simulink model "sampleModel1425"  (R2023a)
settings: Solver=VariableStepAuto  StartTime=0.0  StopTime=10.0  RelTol=1e-3
libraries: hdlsllib x10, simulink x3
settings Model: Creator=user1  LastModifiedBy=user1

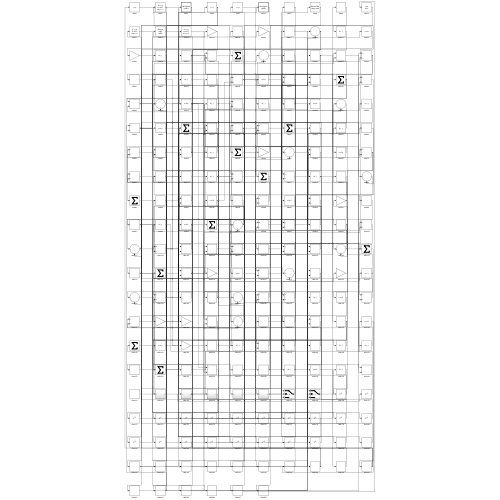
[thumbnail: Simulink's stored preview of the top-level diagram]
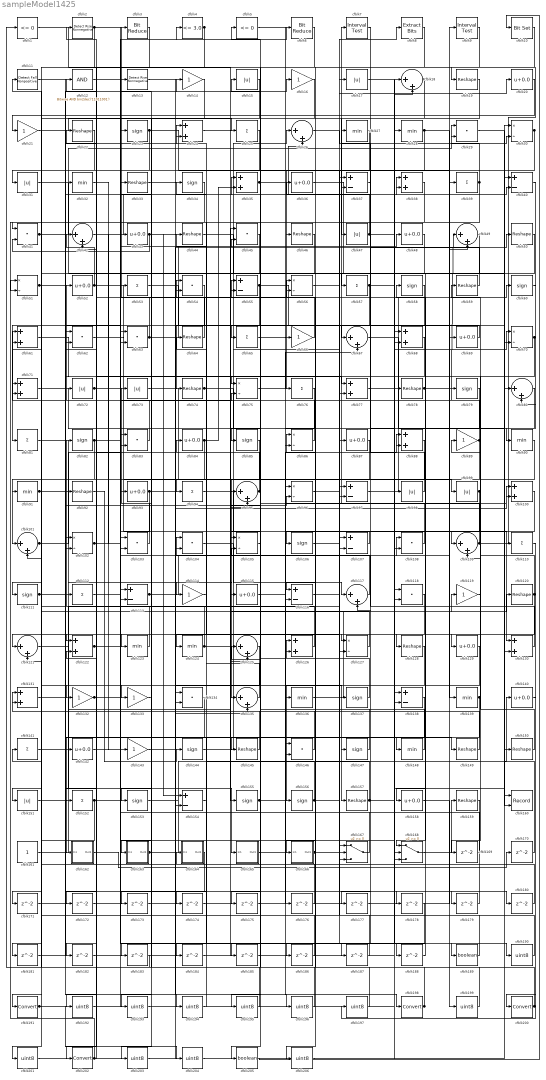
== system sampleModel1425 ==
  cfblk1 : hdlsllib/Logic and Bit Operations/Compare To Zero  relop=<=  OutDataTypeStr=boolean
  cfblk10 : simulink/Logic and Bit Operations/Bit Set  iBit=0
      settings: LibrarySourceBlock=|
      | hdlsllib/Logic and Bit
      | Operations/Bit Set
  cfblk{24,35,38,61,68,71,77,88,100,122,126,130..131} (13 alike) : Sum
  cfblk{18,26,42,49,67,80,95,101,109,117,121,125,135} (13 alike) : Sum  Inputs=|++
  cfblk{30,51,56,70,75,86,96,102,105,127} (10 alike) : Product  Inputs=*/  RndMeth=Zero  SaturateOnIntegerOverflow=on
  cfblk{29,41,45,54,62..63,83,103..104,108,118,134,146} (13 alike) : DotProduct  OutDataTypeStr=Inherit: Inherit via internal rule
  cfblk{23,34,58,60,79,82,85,106,111,137,144,147,153,155..156} (15 alike) : Signum
  cfblk{37,40,55,97,107,113,116,138,154} (9 alike) : Sum  Inputs=+-
  cfblk11 : hdlsllib/Logic and Bit Operations/Detect Fall Nonpositive  vinit=0  OutDataTypeStr=boolean
  cfblk{25,39,53,57,65,76,81,94,110,112,141,152} (12 alike) : Sum  Inputs=+
  cfblk{14,16,21,66,89,114,119,132..133,143} (10 alike) : Gain
  cfblk{20,36,43,48,52,69,84,87,93,115,129,140,142,158} (14 alike) : Bias  Bias=0.0  SaturateOnIntegerOverflow=off
  cfblk12 : simulink/Logic and Bit Operations/Bitwise Operator  logicop=AND  UseBitMask=on  BitMask=bin2dec('11011001')  BitMaskRealWorld=Stored Integer
      settings: LibrarySourceBlock=|
      | hdlsllib/Logic and Bit
      | Operations/Bitwise
      | Operator
  cfblk{19,22,33,44,46,50,59,64,74,78,92,120,128,145,149..150,157,159} (18 alike) : Reshape
  cfblk{27..28,32,90..91,123..124,136,139,148} (10 alike) : MinMax
  cfblk13 : hdlsllib/Logic and Bit Operations/Detect Rise Nonnegative  vinit=0  OutDataTypeStr=boolean
  cfblk{15,17,31,47,72..73,98..99,151} (9 alike) : Abs  SaturateOnIntegerOverflow=off
  cfblk160 : Record  FileSettingsInternal="{\"entries\":[{\"content\":{\"excelSettings\":{\"content\":{},\"type\":\"Streamout.ExcelSettings\"}},\"type\":\"Streamout.FileSettingStorage\",\"uuid\":\"\"}],\"packageUris\":[\"http:\\/\\/schema.mathworks.com\\/mf0\\/streamout_blocks\\/R2020a\"],\"version\":\"1.0\"}"  Layout=[1 1]  SignalsInternal="{\"entries\":[{\"content\":{\"signals\":[{\"content\":{\"blockPath\":[],\"dimensions\":[1],\"domain\":\"\",\"lineColor\":\"#a2142f\",\"plots\":[1],\"port\":1,\"signalID\":401,\"signalName\":\"XY Graph:1\"},\"type\":\"RecordBlkView.Signal\",\"uuid\":\"\"},{\"content\":{\"blockPath\":[],\"dimensions\":[1],\"domain\":\"\",\"lineColor\":\"#139fff\",\"plots\":[1],\"port\":2,\"signalID\":404,\"signalName\":\"XY Graph:2\"},\"type\":\"RecordBlkView.Signal\",\"uuid\":\"\"}]},\"type\":\"RecordBlkView.InputSignals\",\"uuid\":\"\"}],\"packageUris\":[\"http:\\/\\/schema.mathworks.com\\/mf0\\/streamout_blocks\\/R2020a\"],\"version\":\"1.0\"}"  VisualizationBindings="{\"xyplotplugin\":{\"info\":[{\"series\":[{\"bindingParametersList\":[{\"parameter\":\"X-Axis\",\"signalID\":401,\"signalName\":\"XY Graph:1\"},{\"parameter\":\"Y-Axis\",\"signalID\":404,\"signalName\":\"XY Graph:2\"}],\"seriesID\":26922}],\"subplotID\":1}]}}"  CompatibilityTag=XY  st=-1
  cfblk161 : Constant  SampleTime=-1
  cfblk162 : Subsystem
      settings: LibrarySourceBlock=|
      | hdlsllib/Ports &
      | Subsystems/Subsystem
  cfblk163 : Subsystem
      settings: LibrarySourceBlock=|
      | hdlsllib/Ports &
      | Subsystems/Subsystem
  cfblk164 : Subsystem
      settings: LibrarySourceBlock=|
      | hdlsllib/Ports &
      | Subsystems/Subsystem
  cfblk165 : Subsystem
      settings: LibrarySourceBlock=|
      | hdlsllib/Ports &
      | Subsystems/Subsystem
  cfblk166 : Subsystem
      settings: LibrarySourceBlock=|
      | hdlsllib/Ports &
      | Subsystems/Subsystem
  cfblk167 : Switch  SaturateOnIntegerOverflow=off  InputSameDT=off
  cfblk168 : Switch  SaturateOnIntegerOverflow=off  InputSameDT=off
  cfblk{169..188} (20 alike) : Delay  SampleTime=1
  cfblk189 : DataTypeConversion  OutDataTypeStr=boolean  SaturateOnIntegerOverflow=off  RndMeth=Floor
  cfblk{190,192..197,199,201,203..204,206} (12 alike) : DataTypeConversion  OutDataTypeStr=uint8  SaturateOnIntegerOverflow=off  RndMeth=Floor
  cfblk{191,198,200,202} (4 alike) : DataTypeConversion  SaturateOnIntegerOverflow=off  RndMeth=Floor
  cfblk2 : hdlsllib/Logic and Bit Operations/Detect Rise Nonnegative  vinit=0  OutDataTypeStr=boolean
  cfblk205 : DataTypeConversion  OutDataTypeStr=boolean  SaturateOnIntegerOverflow=off  RndMeth=Floor
  cfblk3 : hdlsllib/Logic and Bit Operations/Bit Reduce  mode=AND
  cfblk4 : hdlsllib/Logic and Bit Operations/Compare To Constant  relop=<=  const=3.0  OutDataTypeStr=boolean
  cfblk5 : hdlsllib/Logic and Bit Operations/Compare To Zero  relop=<=  OutDataTypeStr=boolean
  cfblk6 : hdlsllib/Logic and Bit Operations/Bit Reduce  mode=AND
  cfblk7 : hdlsllib/Logic and Bit Operations/Interval Test  IntervalClosedRight=on  uplimit=0.5  IntervalClosedLeft=on  lowlimit=-0.5  OutDataTypeStr=boolean
  cfblk8 : simulink/Logic and Bit Operations/Extract Bits  bitsToExtract=Upper half  numBits=8  bitIdxRange=[0 7]  outScalingMode=Preserve fixed-point scaling
      settings: LibrarySourceBlock=|
      | hdlsllib/Logic and Bit
      | Operations/Extract Bits
  cfblk9 : hdlsllib/Logic and Bit Operations/Interval Test  IntervalClosedRight=on  uplimit=0.5  IntervalClosedLeft=on  lowlimit=-0.5  OutDataTypeStr=boolean
  wires:
  cfblk128/1 -> cfblk157/1
  cfblk144/1 -> cfblk26/1
  cfblk21/1 -> cfblk25/1
  cfblk20/1 -> cfblk21/1
  cfblk166/1(Out1) -> cfblk38/1, cfblk188/1
  cfblk36/1 -> cfblk158/1
  cfblk109/1 -> cfblk19/1, cfblk83/2
  cfblk27/1 -> cfblk31/1
  cfblk32/1 -> cfblk143/1
  cfblk130/1 -> cfblk104/1
  cfblk81/1 -> cfblk165/1(In1)
  cfblk64/1 -> cfblk3/1
  cfblk92/1 -> cfblk144/1
  cfblk87/1 -> cfblk135/1
  cfblk73/1 -> cfblk99/1
  cfblk108/1 -> cfblk7/1
  cfblk123/1 -> cfblk82/1
  cfblk78/1 -> cfblk49/1, cfblk168/1
  cfblk120/1 -> cfblk128/1, cfblk79/1
  cfblk104/1 -> cfblk117/1
  cfblk113/1 -> cfblk9/1, cfblk127/2
  cfblk47/1 -> cfblk36/1, cfblk189/1
  cfblk69/1 -> cfblk65/1
  cfblk18/1 -> cfblk47/1, cfblk193/1
  cfblk147/1 -> cfblk86/1
  cfblk99/1 -> cfblk138/2, cfblk169/1
  cfblk143/1 -> cfblk50/1
  cfblk114/1 -> cfblk44/1
  cfblk70/1 -> cfblk117/2, cfblk129/1
  cfblk153/1 -> cfblk140/1
  cfblk121/1 -> cfblk148/1
  cfblk157/1 -> cfblk70/1, cfblk126/1
  cfblk35/1 -> cfblk26/2, cfblk38/2
  cfblk97/1 -> cfblk39/1
  cfblk54/1 -> cfblk74/1
  cfblk58/1 -> cfblk166/1(In1)
  cfblk139/1 -> cfblk184/1, cfblk195/1
  cfblk149/1 -> cfblk131/1
  cfblk68/1 -> cfblk202/1
  cfblk19/1 -> cfblk105/1
  cfblk129/1 -> cfblk156/1
  cfblk55/1 -> cfblk81/1, cfblk85/1, cfblk108/2
  cfblk161/1 -> cfblk17/1
  cfblk49/1 -> cfblk132/1
  cfblk80/1 -> cfblk147/1
  cfblk84/1 -> cfblk163/1(In1), cfblk35/2
  cfblk41/1 -> cfblk29/1, cfblk75/1
  cfblk116/1 -> cfblk20/1
  cfblk61/1 -> cfblk77/1
  cfblk156/1 -> cfblk87/1, cfblk56/2, cfblk24/2
  cfblk127/1 -> cfblk61/1
  cfblk110/1 -> cfblk200/1
  cfblk71/1 -> cfblk136/1
  cfblk28/1 -> cfblk69/1, cfblk167/3, cfblk177/1
  cfblk15/1 -> cfblk123/1
  cfblk56/1 -> cfblk167/1
  cfblk30/1 -> cfblk76/1, cfblk175/1
  cfblk14/1 -> cfblk121/1
  cfblk63/1 -> cfblk48/1, cfblk2/1
  cfblk77/1 -> cfblk30/1
  cfblk136/1 -> cfblk119/1
  cfblk101/1 -> cfblk23/1, cfblk71/2
  cfblk86/1 -> cfblk61/2
  cfblk165/1(Out1) -> cfblk88/1
  cfblk17/1 -> cfblk109/1
  cfblk62/1 -> cfblk130/1
  cfblk168/1 -> cfblk159/1
  cfblk25/1 -> cfblk111/1
  cfblk39/1 -> cfblk124/1, cfblk51/2, cfblk29/2
  cfblk142/1 -> cfblk16/1
  cfblk112/1 -> cfblk60/1
  cfblk152/1 -> cfblk45/2, cfblk168/3, cfblk201/1
  cfblk91/1 -> cfblk115/1, cfblk179/1
  cfblk52/1 -> cfblk97/2, cfblk42/1
  cfblk103/1 -> cfblk73/1
  cfblk72/1 -> cfblk122/1, cfblk54/2, cfblk185/1
  cfblk83/1 -> cfblk52/1
  cfblk88/1 -> cfblk103/2
  cfblk107/1 -> cfblk106/1
  cfblk126/1 -> cfblk71/1
  cfblk89/1 -> cfblk34/1, cfblk101/1
  cfblk122/1 -> cfblk6/1, cfblk56/1
  cfblk163/1(Out1) -> cfblk45/1, cfblk100/2
  cfblk145/1 -> cfblk22/1
  cfblk117/1 -> cfblk64/1
  cfblk8/1 -> cfblk46/1
  cfblk43/1 -> cfblk67/1, cfblk154/1, cfblk95/1, cfblk41/2, cfblk135/2
  cfblk53/1 -> cfblk80/1
  cfblk7/1 -> cfblk57/1
  cfblk24/1 -> cfblk146/1
  cfblk125/1 -> cfblk151/1
  cfblk155/1 -> cfblk125/1, cfblk100/1
  cfblk38/1 -> cfblk146/2
  cfblk75/1 -> cfblk67/2
  cfblk151/1 -> cfblk96/2
  cfblk31/1 -> cfblk86/2
  cfblk100/1 -> cfblk116/1
  cfblk96/1 -> cfblk107/2
  cfblk60/1 -> cfblk80/2
  cfblk119/1 -> cfblk59/1
  cfblk67/1 -> cfblk160/1
  cfblk131/1 -> cfblk32/1
  cfblk82/1 -> cfblk75/2, cfblk181/1
  cfblk74/1 -> cfblk8/1, cfblk98/1
  cfblk37/1 -> cfblk127/1
  cfblk1/1 -> cfblk155/1
  cfblk134/1 -> cfblk162/1(In1)
  cfblk111/1 -> cfblk149/1, cfblk154/2
  cfblk29/1 -> cfblk130/2
  cfblk23/1 -> cfblk78/1, cfblk139/1, cfblk62/2
  cfblk137/1 -> cfblk83/1
  cfblk4/1 -> cfblk42/2, cfblk192/1
  cfblk124/1 -> cfblk62/1, cfblk120/1
  cfblk94/1 -> cfblk150/1
  cfblk45/1 -> cfblk121/2
  cfblk118/1 -> cfblk191/1
  cfblk159/1 -> cfblk164/1(In1)
  cfblk57/1 -> cfblk77/2, cfblk160/2, cfblk66/1
  cfblk59/1 -> cfblk27/1
  cfblk50/1 -> cfblk142/1
  cfblk26/1 -> cfblk30/2
  cfblk34/1 -> cfblk41/1
  cfblk9/1 -> cfblk145/1
  cfblk42/1 -> cfblk18/2
  cfblk105/1 -> cfblk55/1
  cfblk148/1 -> cfblk92/1
  cfblk76/1 -> cfblk116/2
  cfblk150/1 -> cfblk89/1
  cfblk93/1 -> cfblk134/1, cfblk113/2
  cfblk95/1 -> cfblk94/1, cfblk72/1
  cfblk16/1 -> cfblk133/1
  cfblk102/1 -> cfblk114/1, cfblk43/1, cfblk186/1
  cfblk106/1 -> cfblk40/2
  cfblk167/1 -> cfblk54/1
  cfblk146/1 -> cfblk131/2
  cfblk138/1 -> cfblk153/1
  cfblk98/1 -> cfblk37/2
  cfblk33/1 -> cfblk137/1
  cfblk40/1 -> cfblk90/1
  cfblk2/1 -> cfblk167/2, cfblk91/1
  cfblk5/1 -> cfblk198/1
  cfblk44/1 -> cfblk70/2
  cfblk85/1 -> cfblk152/1
  cfblk51/1 -> cfblk14/1, cfblk35/1, cfblk63/2, cfblk24/1
  cfblk22/1 -> cfblk102/2
  cfblk90/1 -> cfblk109/2
  cfblk135/1 -> cfblk104/2
  cfblk66/1 -> cfblk53/1
  cfblk132/1 -> cfblk4/1, cfblk108/1
  cfblk169/1 -> cfblk103/1
  cfblk162/1(Out1) -> cfblk170/1
  cfblk170/1 -> cfblk40/1
  cfblk3/1 -> cfblk171/1
  cfblk171/1 -> cfblk107/1
  cfblk46/1 -> cfblk172/1
  cfblk172/1 -> cfblk96/1
  cfblk133/1 -> cfblk173/1
  cfblk173/1 -> cfblk37/1
  cfblk154/1 -> cfblk174/1
  cfblk174/1 -> cfblk125/2
  cfblk175/1 -> cfblk138/1
  cfblk65/1 -> cfblk176/1
  cfblk176/1 -> cfblk113/1
  cfblk177/1 -> cfblk49/2
  cfblk115/1 -> cfblk178/1
  cfblk179/1 -> cfblk101/2
  cfblk141/1 -> cfblk180/1
  cfblk180/1 -> cfblk88/2
  cfblk181/1 -> cfblk102/1
  cfblk6/1 -> cfblk182/1
  cfblk182/1 -> cfblk18/1
  cfblk164/1(Out1) -> cfblk183/1
  cfblk183/1 -> cfblk1/1
  cfblk184/1 -> cfblk95/2
  cfblk185/1 -> cfblk105/2
  cfblk186/1 -> cfblk55/2
  cfblk79/1 -> cfblk187/1
  cfblk187/1 -> cfblk97/1
  cfblk188/1 -> cfblk58/1
  cfblk189/1 -> cfblk12/1
  cfblk12/1 -> cfblk190/1
  cfblk190/1 -> cfblk141/1
  cfblk191/1 -> cfblk63/1, cfblk204/1
  cfblk192/1 -> cfblk118/1
  cfblk193/1 -> cfblk118/2
  cfblk11/1 -> cfblk194/1
  cfblk194/1 -> cfblk84/1
  cfblk195/1 -> cfblk11/1
  cfblk13/1 -> cfblk196/1
  cfblk196/1 -> cfblk93/1
  cfblk140/1 -> cfblk197/1
  cfblk197/1 -> cfblk13/1
  cfblk198/1 -> cfblk122/2, cfblk15/1
  cfblk158/1 -> cfblk199/1
  cfblk199/1 -> cfblk5/1
  cfblk200/1 -> cfblk168/2, cfblk126/2, cfblk33/1
  cfblk201/1 -> cfblk110/1
  cfblk202/1 -> cfblk51/1, cfblk134/2, cfblk112/1
  cfblk178/1 -> cfblk203/1
  cfblk203/1 -> cfblk68/1
  cfblk204/1 -> cfblk68/2
  cfblk48/1 -> cfblk205/1
  cfblk205/1 -> cfblk10/1
  cfblk10/1 -> cfblk206/1
  cfblk206/1 -> cfblk28/1

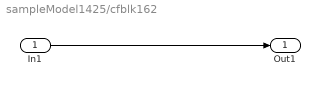
== system sampleModel1425/cfblk162 ==
  In1 : Inport
  Out1 : Outport
  wires:
  In1/1 -> Out1/1

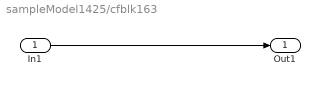
== system sampleModel1425/cfblk163 ==
  In1 : Inport
  Out1 : Outport
  wires:
  In1/1 -> Out1/1

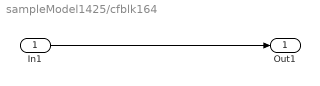
== system sampleModel1425/cfblk164 ==
  In1 : Inport
  Out1 : Outport
  wires:
  In1/1 -> Out1/1

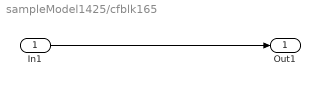
== system sampleModel1425/cfblk165 ==
  In1 : Inport
  Out1 : Outport
  wires:
  In1/1 -> Out1/1

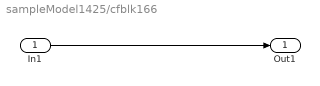
== system sampleModel1425/cfblk166 ==
  In1 : Inport
  Out1 : Outport
  wires:
  In1/1 -> Out1/1
